simulink model "receiver_overall_v3"  (Simulink 7.5)
settings: Solver=FixedStepDiscrete  SolverMode=SingleTasking  StartTime=0.0  StopTime=(length(simin.signals.values)-1)/Fs  FixedStep=1  RelTol=1e-3
undefined symbols (not defined in the file): Fs
libraries: xbsIndex_r4 x939, symbols x8, dspsigops x2
(part 2 of 9)

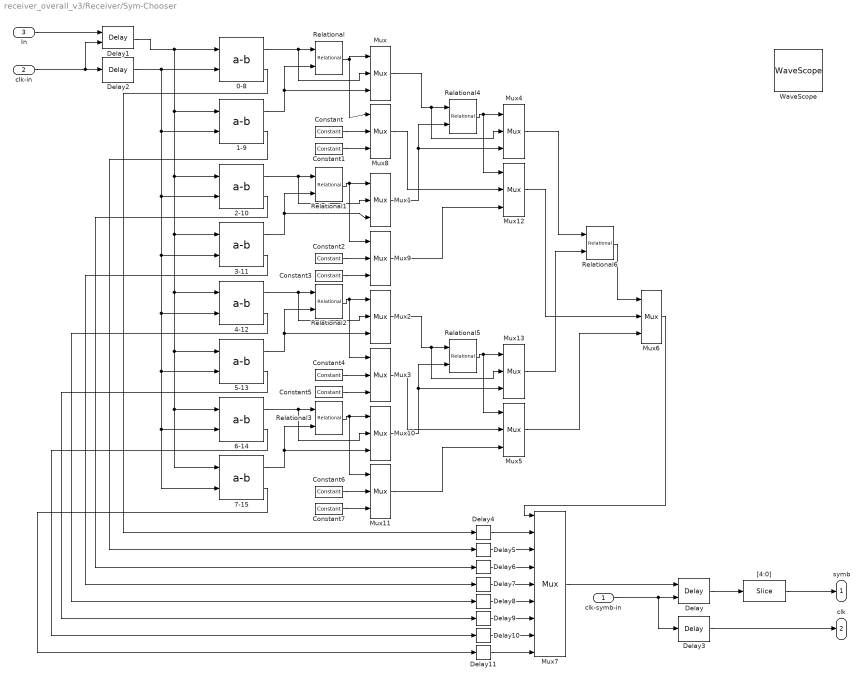
== system receiver_overall_v3/Receiver/Sym-Chooser ==
  clk-symb-in : Inport
  clk-in : Inport  Port=2
  In : Inport  Port=3
  0-8 : symbols/a-b  SystemSampleTime=-1  a=0  b=8  chip_a=1618456172
  1-9 : symbols/a-b  SystemSampleTime=-1  a=1  b=9  chip_a=1309113062
  2-10 : symbols/a-b  SystemSampleTime=-1  a=2  b=10  chip_a=1826650030
  3-11 : symbols/a-b  SystemSampleTime=-1  a=3  b=11  chip_a=1724778362
  4-12 : symbols/a-b  SystemSampleTime=-1  a=4  b=12  chip_a=778887287
  5-13 : symbols/a-b  SystemSampleTime=-1  a=5  b=13  chip_a=2061946375
  6-14 : symbols/a-b  SystemSampleTime=-1  a=6  b=14  chip_a=2007919840
  7-15 : symbols/a-b  SystemSampleTime=-1  a=7  b=15  chip_a=125494990
  Constant : xbsIndex_r4/Constant  arith_type=Unsigned  const=0  n_bits=3  bin_pt=0  explicit_period=off  period=1  equ=P=C  opselect=C  inp2=PCIN>>17  opr=+  inp1=P  carry=CIN  dbl_ovrd=off  block_type=constant
      settings: block_version=12.2
  Constant1 : xbsIndex_r4/Constant  arith_type=Unsigned  const=1  n_bits=3  bin_pt=0  explicit_period=off  period=1  equ=P=C  opselect=C  inp2=PCIN>>17  opr=+  inp1=P  carry=CIN  dbl_ovrd=off  block_type=constant
      settings: block_version=12.2
  Constant2 : xbsIndex_r4/Constant  arith_type=Unsigned  const=2  n_bits=3  bin_pt=0  explicit_period=off  period=1  equ=P=C  opselect=C  inp2=PCIN>>17  opr=+  inp1=P  carry=CIN  dbl_ovrd=off  block_type=constant
      settings: block_version=12.2
  Constant3 : xbsIndex_r4/Constant  arith_type=Unsigned  const=3  n_bits=3  bin_pt=0  explicit_period=off  period=1  equ=P=C  opselect=C  inp2=PCIN>>17  opr=+  inp1=P  carry=CIN  dbl_ovrd=off  block_type=constant
      settings: block_version=12.2
  Constant4 : xbsIndex_r4/Constant  arith_type=Unsigned  const=4  n_bits=3  bin_pt=0  explicit_period=off  period=1  equ=P=C  opselect=C  inp2=PCIN>>17  opr=+  inp1=P  carry=CIN  dbl_ovrd=off  block_type=constant
      settings: block_version=12.2
  Constant5 : xbsIndex_r4/Constant  arith_type=Unsigned  const=5  n_bits=3  bin_pt=0  explicit_period=off  period=1  equ=P=C  opselect=C  inp2=PCIN>>17  opr=+  inp1=P  carry=CIN  dbl_ovrd=off  block_type=constant
      settings: block_version=12.2
  Constant6 : xbsIndex_r4/Constant  arith_type=Unsigned  const=6  n_bits=3  bin_pt=0  explicit_period=off  period=1  equ=P=C  opselect=C  inp2=PCIN>>17  opr=+  inp1=P  carry=CIN  dbl_ovrd=off  block_type=constant
      settings: block_version=12.2
  Constant7 : xbsIndex_r4/Constant  arith_type=Unsigned  const=7  n_bits=3  bin_pt=0  explicit_period=off  period=1  equ=P=C  opselect=C  inp2=PCIN>>17  opr=+  inp1=P  carry=CIN  dbl_ovrd=off  block_type=constant
      settings: block_version=12.2
  Delay : xbsIndex_r4/Delay  en=on  latency=1  dbl_ovrd=off  reg_retiming=off  block_type=delay
      settings: block_version=12.2
  Delay1 : xbsIndex_r4/Delay  en=on  latency=1  dbl_ovrd=off  reg_retiming=off  block_type=delay
      settings: block_version=12.2
  Delay{2..11} (10 alike) : xbsIndex_r4/Delay  en=off  latency=1  dbl_ovrd=off  reg_retiming=off  block_type=delay
      settings: block_version=12.2
  Mux{,1..3,6,8..11} (9 alike) : xbsIndex_r4/Mux  inputs=2  en=off  latency=0  precision=Full  arith_type=Unsigned  n_bits=16  bin_pt=14  quantization=Truncate  overflow=Wrap  dbl_ovrd=off  block_type=mux
      settings: block_version=12.2
  Mux{4..5,12..13} (4 alike) : xbsIndex_r4/Mux  inputs=2  en=off  latency=1  precision=Full  arith_type=Unsigned  n_bits=16  bin_pt=14  quantization=Truncate  overflow=Wrap  dbl_ovrd=off  block_type=mux
      settings: block_version=12.2
  Mux7 : xbsIndex_r4/Mux  inputs=8  en=off  latency=0  precision=Full  arith_type=Unsigned  n_bits=16  bin_pt=14  quantization=Truncate  overflow=Wrap  dbl_ovrd=off  block_type=mux
      settings: block_version=12.2
  Relational{,1..6} (7 alike) : xbsIndex_r4/Relational  mode=a<b  en=off  latency=0  dbl_ovrd=off  block_type=relational
      settings: block_version=12.2
  WaveScope : xbsIndex_r4/WaveScope  block_type=wavescope
      settings: block_version=12.2
  "[4:0]" : xbsIndex_r4/Slice  nbits=4  boolean_output=off  mode=Lower Bit Location + Width  bit1=0  base1=MSB of Input  bit0=0  base0=LSB of Input  dbl_ovrd=off  block_type=slice
      settings: block_version=12.1
  symb : Outport
  clk : Outport  Port=2
  wires:
  "[4:0]"/1 -> symb/1
  Delay1/1 -> 0-8/1, 1-9/1, 2-10/1, 3-11/1, 4-12/1, 5-13/1, 7-15/1, 6-14/1
  Relational/1 -> Mux/1, Mux8/1
  0-8/1 -> Relational/1, Mux/2
  1-9/1 -> Relational/2, Mux/3
  0-8/2 -> Delay4/1
  1-9/2 -> Delay5/1
  2-10/2 -> Delay6/1
  3-11/2 -> Delay7/1
  4-12/2 -> Delay8/1
  5-13/2 -> Delay9/1
  6-14/2 -> Delay10/1
  7-15/2 -> Delay11/1
  Constant/1 -> Mux8/2
  Constant1/1 -> Mux8/3
  Relational1/1 -> Mux1/1, Mux9/1
  2-10/1 -> Relational1/1, Mux1/2
  3-11/1 -> Relational1/2, Mux1/3
  Constant2/1 -> Mux9/2
  Constant3/1 -> Mux9/3
  Relational2/1 -> Mux2/1, Mux3/1
  4-12/1 -> Relational2/1, Mux2/2
  5-13/1 -> Mux2/3, Relational2/2
  Constant4/1 -> Mux3/2
  Constant5/1 -> Mux3/3
  Relational3/1 -> Mux10/1, Mux11/1
  6-14/1 -> Relational3/1, Mux10/2
  7-15/1 -> Relational3/2, Mux10/3
  Constant6/1 -> Mux11/2
  Constant7/1 -> Mux11/3
  Relational4/1 -> Mux4/1, Mux12/1
  Mux/1 -> Relational4/1, Mux4/2
  Mux1/1 -> Relational4/2, Mux4/3
  Mux8/1 -> Mux12/2
  Mux9/1 -> Mux12/3
  Relational5/1 -> Mux13/1, Mux5/1
  Mux2/1 -> Relational5/1, Mux13/2
  Mux10/1 -> Relational5/2, Mux13/3
  Mux3/1 -> Mux5/2
  Mux11/1 -> Mux5/3
  Relational6/1 -> Mux6/1
  Mux4/1 -> Relational6/1
  Mux13/1 -> Relational6/2
  Mux12/1 -> Mux6/2
  Mux5/1 -> Mux6/3
  clk-in/1 -> Delay1/2, Delay2/1
  Mux7/1 -> Delay/1
  Delay/1 -> "[4:0]"/1
  clk-symb-in/1 -> Delay/2, Delay3/1
  Mux6/1 -> Mux7/1
  In/1 -> Delay1/1
  Delay4/1 -> Mux7/2
  Delay5/1 -> Mux7/3
  Delay6/1 -> Mux7/4
  Delay7/1 -> Mux7/5
  Delay8/1 -> Mux7/6
  Delay9/1 -> Mux7/7
  Delay10/1 -> Mux7/8
  Delay11/1 -> Mux7/9
  Delay2/1 -> 0-8/2, 6-14/2, 7-15/2, 5-13/2, 4-12/2, 3-11/2, 2-10/2, 1-9/2
  Delay3/1 -> clk/1

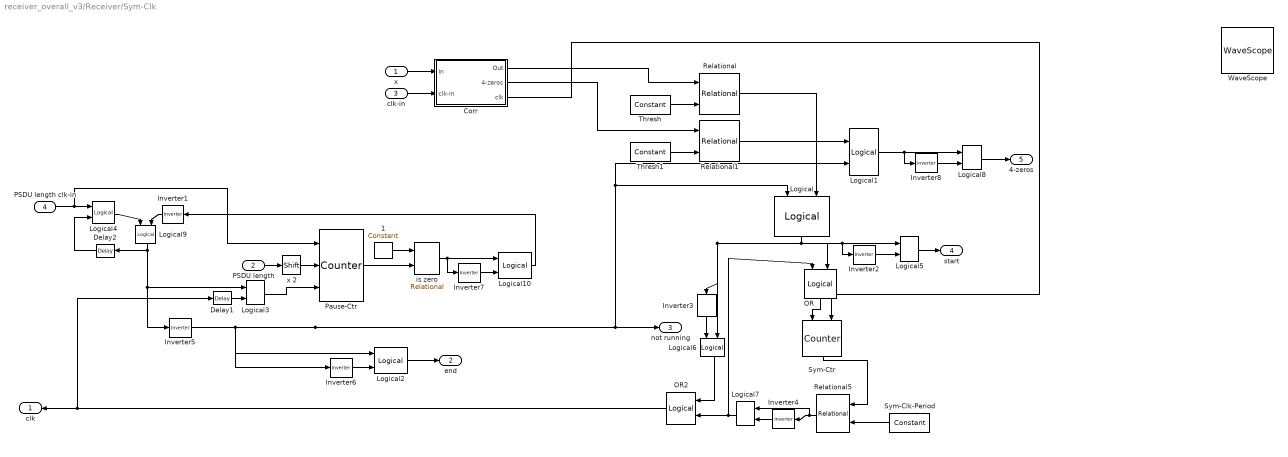
== system receiver_overall_v3/Receiver/Sym-Clk ==
  x : Inport
  PSDU length : Inport  Port=2  OutDataType=fixdt(1, 16)  OutScaling=2^0
  clk-in : Inport  Port=3
  PSDU length clk-in : Inport  Port=4  OutDataType=fixdt(1, 16)  OutScaling=2^0
  1 : xbsIndex_r4/Constant  arith_type=Unsigned  const=0  n_bits=1  bin_pt=0  explicit_period=off  period=1  equ=P=C  opselect=C  inp2=PCIN>>17  opr=+  inp1=P  carry=CIN  dbl_ovrd=off  block_type=constant
      settings: block_version=12.1
  Corr : Subsystem
  Delay1 : xbsIndex_r4/Delay  en=off  latency=3  dbl_ovrd=off  reg_retiming=off  block_type=delay
      settings: block_version=12.2
  Delay2 : xbsIndex_r4/Delay  en=off  latency=1  dbl_ovrd=off  reg_retiming=off  block_type=delay
      settings: block_version=12.2
  Inverter{1..4,6..8} (7 alike) : xbsIndex_r4/Inverter  en=off  latency=1  dbl_ovrd=off  block_type=inv
      settings: block_version=12.2
  Inverter5 : xbsIndex_r4/Inverter  en=off  latency=0  dbl_ovrd=off  block_type=inv
      settings: block_version=12.2
  Logical{,1..3,5..10} (10 alike) : xbsIndex_r4/Logical  logical_function=AND  inputs=2  en=off  latency=0  precision=Full  arith_type=Unsigned  n_bits=16  bin_pt=0  align_bp=on  dbl_ovrd=off  block_type=logical
      Logical settings: xl_area=[1 0 0 2 0 0 0]  block_version=12.1
      Logical1 settings: xl_area=[1 0 0 2 0 0 0]  block_version=12.1
      Logical10 settings: block_version=12.2
      Logical2 settings: block_version=12.2
      Logical3 settings: block_version=12.2
      Logical5 settings: block_version=12.2
      Logical6 settings: block_version=12.2
      Logical7 settings: block_version=12.2
      Logical8 settings: block_version=12.2
      Logical9 settings: block_version=12.2
  Logical4 : xbsIndex_r4/Logical  logical_function=OR  inputs=2  en=off  latency=0  precision=Full  arith_type=Unsigned  n_bits=16  bin_pt=0  align_bp=on  dbl_ovrd=off  block_type=logical
      settings: block_version=12.2
  OR : xbsIndex_r4/Logical  logical_function=OR  inputs=2  en=off  latency=0  precision=Full  arith_type=Unsigned  n_bits=16  bin_pt=0  align_bp=on  dbl_ovrd=off  block_type=logical
      settings: xl_area=[1 0 0 1 0 0 0]  block_version=12.1
  OR2 : xbsIndex_r4/Logical  logical_function=OR  inputs=2  en=off  latency=0  precision=Full  arith_type=Unsigned  n_bits=16  bin_pt=0  align_bp=on  dbl_ovrd=off  block_type=logical
      settings: xl_area=[1 0 0 1 0 0 0]  block_version=12.1
  Pause-Ctr : xbsIndex_r4/Counter  cnt_type=Free Running  cnt_to=Inf  operation=Down  start_count=0  cnt_by_val=1  arith_type=Unsigned  n_bits=13  bin_pt=0  load_pin=on  rst=off  en=on  explicit_period=off  period=1600  dbl_ovrd=off  use_behavioral_HDL=off  implementation=Fabric  block_type=counter
      settings: block_version=12.2
  Relational : xbsIndex_r4/Relational  mode=a>b  en=off  latency=0  dbl_ovrd=off  block_type=relational
      settings: xl_area=[4 0 0 7 0 0 0]  block_version=12.1
  Relational1 : xbsIndex_r4/Relational  mode=a>b  en=off  latency=0  dbl_ovrd=off  block_type=relational
      settings: xl_area=[4 0 0 7 0 0 0]  block_version=12.1
  Relational5 : xbsIndex_r4/Relational  mode=a=b  en=off  latency=1  dbl_ovrd=off  block_type=relational
      settings: xl_area=[2 0 0 4 0 0 0]  block_version=12.1
  Sym-Clk-Period : xbsIndex_r4/Constant  arith_type=Unsigned  const=32  n_bits=6  bin_pt=0  explicit_period=off  period=1  equ=P=C  opselect=C  inp2=PCIN>>17  opr=+  inp1=P  carry=CIN  dbl_ovrd=off  block_type=constant
      settings: block_version=12.1
  Sym-Ctr : xbsIndex_r4/Counter  cnt_type=Free Running  cnt_to=0  operation=Up  start_count=0  cnt_by_val=1  arith_type=Unsigned  n_bits=8  bin_pt=0  load_pin=off  rst=on  en=on  explicit_period=off  period=1  dbl_ovrd=off  use_behavioral_HDL=off  implementation=Fabric  block_type=counter
      settings: xl_area=[5 8 0 8 0 0 0]  block_version=12.1
  Thresh : xbsIndex_r4/Constant  arith_type=Unsigned  const=80  n_bits=7  bin_pt=0  explicit_period=off  period=1  equ=P=C  opselect=C  inp2=PCIN>>17  opr=+  inp1=P  carry=CIN  dbl_ovrd=off  block_type=constant
      settings: block_version=12.1
  Thresh1 : xbsIndex_r4/Constant  arith_type=Unsigned  const=80  n_bits=7  bin_pt=0  explicit_period=off  period=1  equ=P=C  opselect=C  inp2=PCIN>>17  opr=+  inp1=P  carry=CIN  dbl_ovrd=off  block_type=constant
      settings: block_version=12.1
  WaveScope : xbsIndex_r4/WaveScope  block_type=wavescope
      settings: block_version=12.2
  is zero : xbsIndex_r4/Relational  mode=a=b  en=off  latency=0  dbl_ovrd=off  block_type=relational
      settings: block_version=12.2
  x 2 : xbsIndex_r4/Shift  shift_dir=Left  shift_bits=1  en=off  latency=0  precision=User Defined  arith_type=Unsigned  n_bits=13  bin_pt=0  quantization=Truncate  overflow=Wrap  dbl_ovrd=off  block_type=shift
      settings: block_version=12.2
  clk : Outport  OutDataType=fixdt(1, 16)  OutScaling=2^0
  end : Outport  Port=2  OutDataType=fixdt(1, 16)  OutScaling=2^0
  not running : Outport  Port=3  OutDataType=fixdt(1, 16)  OutScaling=2^0
  start : Outport  Port=4  OutDataType=fixdt(1, 16)  OutScaling=2^0
  4-zeros : Outport  Port=5  OutDataType=fixdt(1, 16)  OutScaling=2^0
  wires:
  Thresh/1 -> Relational/2
  Relational/1 -> Logical/2
  Logical/1 -> OR/2, Logical5/1, Inverter2/1, Inverter3/1, Logical6/2
  x/1 -> Corr/1(In)
  OR/1 -> Sym-Ctr/1
  Inverter5/1 -> not running/1, Logical/1, Logical1/2, Logical2/1, Inverter6/1
  Logical2/1 -> end/1
  Sym-Ctr/1 -> Relational5/1
  Inverter6/1 -> Logical2/2
  Sym-Clk-Period/1 -> Relational5/2
  OR2/1 -> clk/1, Delay1/1
  Thresh1/1 -> Relational1/2
  Relational1/1 -> Logical1/1
  clk-in/1 -> Corr/2(clk-in)
  Corr/2(4-zeros) -> Relational1/1
  Logical5/1 -> start/1
  Inverter2/1 -> Logical5/2
  Corr/1(Out) -> Relational/1
  Corr/3(clk) -> Sym-Ctr/2
  Inverter3/1 -> Logical6/1
  Logical6/1 -> OR2/1
  Inverter4/1 -> Logical7/2
  Relational5/1 -> Inverter4/1, Logical7/1
  Logical7/1 -> OR2/2, OR/1
  Delay2/1 -> Logical4/2
  Logical4/1 -> Logical9/1
  Inverter1/1 -> Logical9/2
  Logical9/1 -> Delay2/1, Logical3/1, Inverter5/1
  x 2/1 -> Pause-Ctr/2
  PSDU length/1 -> x 2/1
  PSDU length clk-in/1 -> Logical4/1, Pause-Ctr/1
  Logical3/1 -> Pause-Ctr/3
  1/1 -> is zero/1
  Pause-Ctr/1 -> is zero/2
  Inverter7/1 -> Logical10/2
  is zero/1 -> Inverter7/1, Logical10/1
  Logical10/1 -> Inverter1/1
  Delay1/1 -> Logical3/2
  Logical1/1 -> Logical8/1, Inverter8/1
  Inverter8/1 -> Logical8/2
  Logical8/1 -> 4-zeros/1

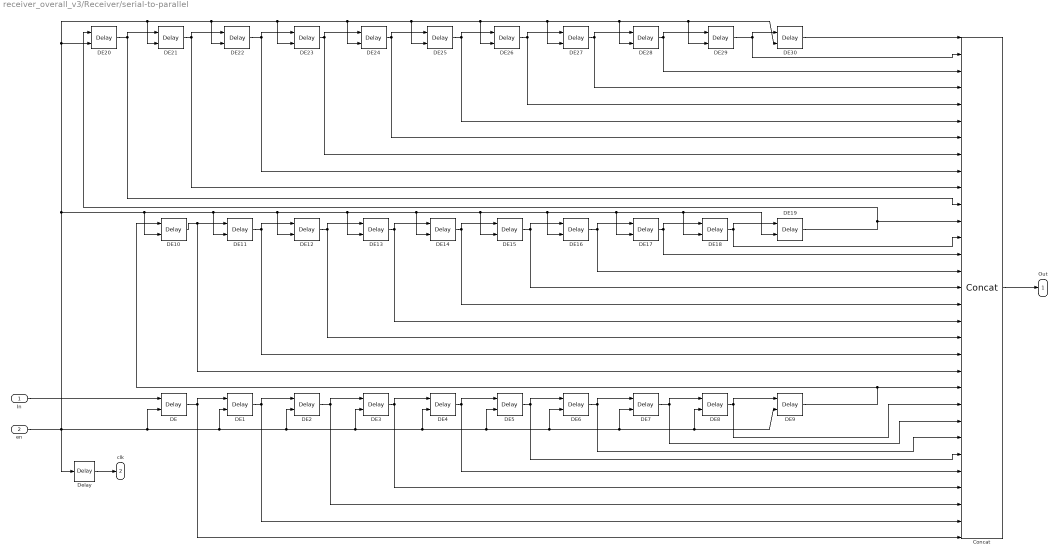
== system receiver_overall_v3/Receiver/serial-to-parallel ==
  In : Inport
  en : Inport  Port=2
  Concat : xbsIndex_r4/Concat  num_inputs=31  dbl_ovrd=off  block_type=concat
      settings: block_version=12.1
  DE{,1..30} (31 alike) : xbsIndex_r4/Delay  en=on  latency=1  dbl_ovrd=off  reg_retiming=off  block_type=delay
      settings: xl_area=[1 1 0 0 0 0 0]  block_version=12.1
  Delay : xbsIndex_r4/Delay  en=off  latency=1  dbl_ovrd=off  reg_retiming=off  block_type=delay
      settings: block_version=12.2
  Out : Outport
  clk : Outport  Port=2
  wires:
  In/1 -> DE/1
  en/1 -> DE20/2, DE21/2, DE22/2, DE23/2, DE24/2, DE25/2, DE26/2, DE27/2, DE28/2, DE30/2, DE29/2, DE19/2, DE18/2, DE17/2, DE16/2, DE15/2, DE14/2, DE13/2, DE12/2, DE11/2, DE10/2, DE1/2, DE2/2, DE3/2, DE4/2, DE5/2, DE6/2, DE7/2, DE8/2, DE9/2, DE/2, Delay/1
  DE/1 -> DE1/1, Concat/31
  DE1/1 -> DE2/1, Concat/30
  DE2/1 -> DE3/1, Concat/29
  DE3/1 -> DE4/1, Concat/28
  DE4/1 -> DE5/1, Concat/27
  DE5/1 -> DE6/1, Concat/26
  DE6/1 -> DE7/1, Concat/25
  DE8/1 -> DE9/1, Concat/23
  DE10/1 -> DE11/1, Concat/21
  DE11/1 -> DE12/1, Concat/20
  DE12/1 -> DE13/1, Concat/19
  DE13/1 -> DE14/1, Concat/18
  DE14/1 -> DE15/1, Concat/17
  DE15/1 -> DE16/1, Concat/16
  DE16/1 -> DE17/1, Concat/15
  DE17/1 -> DE18/1, Concat/14
  DE18/1 -> DE19/1, Concat/13
  DE20/1 -> DE21/1, Concat/11
  DE21/1 -> DE22/1, Concat/10
  DE22/1 -> DE23/1, Concat/9
  DE23/1 -> DE24/1, Concat/8
  DE24/1 -> DE25/1, Concat/7
  DE25/1 -> DE26/1, Concat/6
  DE26/1 -> DE27/1, Concat/5
  DE27/1 -> DE28/1, Concat/4
  DE28/1 -> DE29/1, Concat/3
  DE7/1 -> DE8/1, Concat/24
  DE29/1 -> DE30/1, Concat/2
  DE30/1 -> Concat/1
  DE19/1 -> Concat/12, DE20/1
  DE9/1 -> Concat/22, DE10/1
  Concat/1 -> Out/1
  Delay/1 -> clk/1

== system receiver_overall_v3/Receiver/to octet ==
  In : Inport
  clk-in : Inport  Port=2
  Concat : xbsIndex_r4/Concat  num_inputs=2  dbl_ovrd=off  block_type=concat
      settings: block_version=12.2
  Delay : xbsIndex_r4/Delay  en=on  latency=1  dbl_ovrd=off  reg_retiming=off  block_type=delay
      settings: block_version=12.2
  Delay1 : xbsIndex_r4/Delay  en=off  latency=1  dbl_ovrd=off  reg_retiming=off  block_type=delay
      settings: block_version=12.2
  Delay2 : xbsIndex_r4/Delay  en=off  latency=1  dbl_ovrd=off  reg_retiming=off  block_type=delay
      settings: block_version=12.2
  data : Outport
  clk : Outport  Port=2
  wires:
  Concat/1 -> data/1
  In/1 -> Delay1/1
  Delay1/1 -> Delay/1, Concat/1
  clk-in/1 -> Delay/2, Delay2/1
  Delay/1 -> Concat/2
  Delay2/1 -> clk/1

== system receiver_overall_v3/Receiver/FM demod/AGC ==
  I : Inport
  Q : Inport  Port=2
  CORDIC DIVIDER : Subsystem  mask(Xilinx CORDIC Divider){stages=8, num_width=22, num_binpt=19, pipeline_x=[1 1 1 1 1 1 1 1], prev_stages=8, pipeline=[1  1  1  1  1  1  1  1], prev_bits=21}
      mask prompts: stages "Number of Processing Elements (integer value starting from 1)"; num_width "X, Y, Data Width"; num_binpt "X,Y Binary Point Position"; pipeline_x "Latency for each Processing Element [1 0 0 1]"; prev_stages "Previous Number of Stages"; pipeline "Previous Pipeline Value"; prev_bits "Previous Number of Bits"
      mask help: This design implements a divider circuit using a fully parallel CORDIC (COordinate Rotation DIgital Computer) algorithm in linear vectoring mode with pre and post compensation. Using pre and post compensation techniques, this design can compute any arbitrary ratio y/x.
      mask init:
      | [bg,fg] = xlcmap('XBlock',0);
      | iPos = get_param(gcb,'Position');
      | iWidth=iPos(3)-iPos(1); iHeight=iPos(4)-iPos(2);
      | iCx=iWidth/2;
      | iCy=iHeight/2;
      | [logoX, logoY] = xlogo(iPos);
      | sav_gcb=gcb;
      | stages = round(sum(abs(stages)));
      | if (stages == 0)
      | 	stages = prev_stages;
      | end
      | x = zeros(1,stages);
      | pipe_size = max(size(pipeline_x));
      | if pipe_size >= stages
      | 	x(1,1:stages) = pipeline_x(1,1:stages);
      | else
      | 	x(1,1:pipe_size) = pipeline_x(1,1:pipe_size);
      | end
      | 
      | num_width = round(sum(abs(num_width)));
      | if (num_width < 2)
      | 	num_width = prev_bits;
      | end
      | 
      | if ((num_width-1) ~=prev_bits)
      |     % Draw the Normalization X Stage
      |     norm_x = find_system(sav_gcb, 'lookUnderMasks', 'all', 'FollowLinks','on','masktype', 'Normalize X');
      | 	a=find_system(norm_x{1}, 'lookUnderMasks', 'all', 'FollowLinks','on','masktype', 'Normalize Shift Stage');
      | 	for i= 2:length(a)
      | 		for j=1:3
      | 		    delete_line(norm_x{1}, ['Shift' int2str(i-1) '/' int2str(j)], ['Shift' int2str(i) '/' int2str(j)]);
      | 		end
      | 	end
      | 	delete_line(norm_x{1}, ['Shift' int2str(length(a)) '/1'],'norm/1');
      | 	delete_line(norm_x{1}, ['Shift' int2str(length(a)) '/2'],'shift/1');
      | 	delete_line(norm_x{1}, ['Shift' int2str(length(a)) '/3'],'Terminator1/1');
      | 	
      | 	for i=2:length(a)
      |       delete_block(a{i});
      | 	end
      | 	for i=2:(num_width-1),
      |         add_block([norm_x{1} '/Shift1'], [norm_x{1} '/Shift' int2str(i)],'position',[150+(i-1)*125, 70, 205+(i-1)*125, 130]);
      | 	end
      |     set_param([norm_x{1} '/' 'norm'], 'Position', [150+i*125, 72, 180+i*125, 86]);
      |     set_param([norm_x{1} '/' 'shift'], 'Position', [210+i*125, 92, 225+i*125, 108]);
      |     set_param([norm_x{1} '/' 'Terminator1'], 'Position', [240+i*125, 113, 270+i*125, 127]);
      |     for i= 2:(num_width-1)
      | 		for j=1:3
      | 		    add_line(norm_x{1}, ['Shift' int2str(i-1) '/' int2str(j)], ['Shift' int2str(i) '/' int2str(j)]);
      | 		end
      | 	end
      |     add_line(norm_x{1}, ['Shift' int2str((num_width-1)) '/1'],'norm/1');
      | 	add_line(norm_x{1}, ['Shift' int2str((num_width-1)) '/2'],'shift/1');
      | 	add_line(norm_x{1}, ['Shift' int2str((num_width-1)) '/3'],'Terminator1/1');
      |     
      |     % Draw the Normalization Y Stage
      |     norm_y = find_system(sav_gcb, 'lookUnderMasks', 'all', 'FollowLinks','on','masktype', 'Normalize Y');
      | 	a=find_system(norm_y{1}, 'lookUnderMasks', 'all', 'FollowLinks','on','masktype', 'Normalize Shift Stage');
      | 	for i= 2:length(a)
      | 		for j=1:3
      | 		    delete_line(norm_y{1}, ['Shift' int2str(i-1) '/' int2str(j)], ['Shift' int2str(i) '/' int2str(j)]);
      | 		end
      | 	end
      | 	delete_line(norm_y{1}, ['Shift' int2str(length(a)) '/1'],'norm/1');
      | 	delete_line(norm_y{1}, ['Shift' int2str(length(a)) '/2'],'shift/1');
      | 	delete_line(norm_y{1}, ['Shift' int2str(length(a)) '/3'],'Terminator1/1');
      | 	
      | 	for i=2:length(a)
      |       delete_block(a{i});
      | 	end
      | 	for i=2:(num_width-1)
      |         add_block([norm_y{1} '/Shift1'], [norm_y{1} '/Shift' int2str(i)],'position',[150+(i-1)*125, 70, 205+(i-1)*125, 130]);
      | 	end
      |     set_param([norm_y{1} '/' 'norm'], 'Position', [150+i*125, 72, 180+i*125, 86]);
      |     set_param([norm_y{1} '/' 'shift'], 'Position', [210+i*125, 92, 225+i*125, 108]);
      |     set_param([norm_y{1} '/' 'Terminator1'], 'Position', [240+i*125, 113, 270+i*125, 127]);
      |     for i= 2:(num_width-1)
      | 		for j=1:3
      | 		    add_line(norm_y{1}, ['Shift' int2str(i-1) '/' int2str(j)], ['Shift' int2str(i) '/' int2str(j)]);
      | 		end
      | 	end
      |     add_line(norm_y{1}, ['Shift' int2str((num_width-1)) '/1'],'norm/1');
      | 	add_line(norm_y{1}, ['Shift' int2str((num_width-1)) '/2'],'shift/1');
      | 	add_line(norm_y{1}, ['Shift' int2str((num_width-1)) '/3'],'Terminator1/1');
      | 	find_system(sav_gcb, 'lookUnderMasks', 'all', 'FollowLinks', 'on', 'MaskType','Xilinx Multiplexer Block');
      | 	set_param(sav_gcb, 'prev_bits',int2str((num_width-1)));
      | end
      | if (stages ~=prev_stages)
      | 	pipeline=x;
      |     iterative_divider = find_system(sav_gcb, 'lookUnderMasks', 'all', 'FollowLinks','on','masktype', 'CORDIC Iterative Divider');
      |   a=find_system(iterative_divider{1}, 'lookUnderMasks', 'all', 'FollowLinks','on','masktype', 'CORDIC iteration Divider');
      |   for i= 2:length(a)
      |     for j=1:3
      | 	  delete_line(iterative_divider{1}, ['CORDIC PE' int2str(i-1) '/' int2str(j)], ['CORDIC PE' int2str(i) '/' int2str(j)]);
      |     end
      |   end
      |   delete_line(iterative_divider{1}, ['CORDIC PE' int2str(length(a)) '/1'],'Terminator1/1');
      |   delete_line(iterative_divider{1}, ['CORDIC PE' int2str(length(a)) '/2'],'Terminator2/1');
      |   delete_line(iterative_divider{1}, ['CORDIC PE' int2str(length(a)) '/3'],'Z/1');
      |   for i=2:length(a)
      |      delete_block(a{i});
      |   end
      |   for i=2:stages,
      |       add_block([iterative_divider{1} '/CORDIC PE1'], [iterative_divider{1} '/CORDIC PE' int2str(i)], 'ii', int2str(i-1),'pipeline',['pipeline(1,' int2str(i) ')'],'position',[150+(i-1)*125, 70, 205+(i-1)*125, 130]);
      |   end
      |   for i= 2:stages,
      |      for j=1:3
      | 	     add_line(iterative_divider{1}, ['CORDIC PE' int2str(i-1) '/' int2str(j)], ['CORDIC PE' int2str(i) '/' int2str(j)], 'autorouting', 'on');
      |      end
      |   end
      |   set_param([iterative_divider{1} '/' 'Terminator1'], 'Position', [150+stages*125, 72, 180+stages*125, 86]);
      |   set_param([iterative_divider{1} '/' 'Terminator2'], 'Position', [210+stages*125, 92, 225+stages*125, 108]);
      |   set_param([iterative_divider{1} '/' 'Z'], 'Position', [240+stages*125, 113, 270+stages*125, 127]);
      | 
      |   add_line(iterative_divider{1}, ['CORDIC PE' int2str(stages) '/1'], 'Terminator1/1', 'autorouting', 'on');
      |   add_line(iterative_divider{1}, ['CORDIC PE' int2str(stages) '/2'], 'Terminator2/1', 'autorouting', 'on');
      |   add_line(iterative_divider{1}, ['CORDIC PE' int2str(stages) '/3'],'Z/1', 'autorouting', 'on');
      |    % force a "compile" of the constituent constant blocks to
      |    % workaround a data propagation problem
      |    find_system(iterative_divider{1}, 'lookUnderMasks', 'all', 'FollowLinks', 'on', 'MaskType','Xilinx Constant Block');
      |    set_param(sav_gcb, 'prev_stages', int2str(stages));
      |    set_param(sav_gcb, 'pipeline', [ '[' int2str(x) ']']);
      | else
      | 	if (sum(pipeline~=x))
      | 		set_param(sav_gcb, 'pipeline', [ '[' int2str(x) ']']);
      | 	end
      | end
      | 
      | str = sprintf('-%d',sum(x) + num_width + 4);
      settings: CopyFcn=set_param(gcb, 'MaskSelfModifiable', 'on', 'LinkStatus', 'none');
      mask Help: eval('');xlDoc('-book','sysgen','-topic','CORDIC_DIVIDER');
      mask Display:
      | patch([0 iWidth iWidth 0],[0 0 iHeight iHeight] , bg);
      | patch(logoX,logoY , fg);
      | text(iCx-6,iCy,'z');
      | text(iCx,iCy+4,str);
      | port_label('input',1,'x');
      | port_label('input',2,'y');
      | port_label('output',1,'y/x');
      | plot([0 0 iWidth iWidth 0], [0 iHeight iHeight 0 0]);
  Convert : xbsIndex_r4/Convert  arith_type="Signed  (2's comp)"  n_bits=16  bin_pt=14  quantization=Truncate  overflow=Wrap  en=off  latency=0  dbl_ovrd=off  pipeline=off  block_type=convert
      settings: block_version=12.2
  Convert1 : xbsIndex_r4/Convert  arith_type="Signed  (2's comp)"  n_bits=16  bin_pt=14  quantization=Truncate  overflow=Wrap  en=off  latency=0  dbl_ovrd=off  pipeline=off  block_type=convert
      settings: block_version=12.2
  Moving Average : Subsystem
  Mult4 : xbsIndex_r4/Mult  precision=Full  arith_type="Signed  (2's comp)"  n_bits=16  bin_pt=14  quantization=Truncate  overflow=Wrap  en=off  latency=4  dbl_ovrd=off  use_behavioral_HDL=off  opt=Speed  use_embedded=off  optimum_pipeline=on  pipeline=on  use_rpm=on  placement_style=Triangular  block_type=mult
      settings: block_version=12.2
  Mult5 : xbsIndex_r4/Mult  precision=Full  arith_type="Signed  (2's comp)"  n_bits=16  bin_pt=14  quantization=Truncate  overflow=Wrap  en=off  latency=4  dbl_ovrd=off  use_behavioral_HDL=off  opt=Speed  use_embedded=off  optimum_pipeline=on  pipeline=on  use_rpm=on  placement_style=Triangular  block_type=mult
      settings: block_version=12.2
  level estimate : Subsystem
      mask Display:
      | port_label('input',1,'I');
      | port_label('input',2,'Q');
      | port_label('output',1,'\approx sqrt(I^2+Q^2)','texmode','on');
  reference : xbsIndex_r4/Constant  arith_type=Signed (2's comp)  const=1  n_bits=22  bin_pt=19  explicit_period=on  period=1  equ=P=C  opselect=C  inp2=PCIN>>17  opr=+  inp1=P  carry=CIN  dbl_ovrd=off  block_type=constant
      settings: block_version=12.2
  I' : Outport
  Q' : Outport  Port=2
  wires:
  level estimate/1(Out1) -> Moving Average/1(in)
  I/1 -> level estimate/1(In1), Mult4/1
  Q/1 -> level estimate/2(In2), Mult5/2
  Convert/1 -> I'/1
  Convert1/1 -> Q'/1
  reference/1 -> CORDIC DIVIDER/2(y)
  Moving Average/1(short) -> CORDIC DIVIDER/1(x)
  Mult4/1 -> Convert/1
  Mult5/1 -> Convert1/1
  CORDIC DIVIDER/1(div) -> Mult5/1, Mult4/2

== system receiver_overall_v3/Receiver/FM demod/CORDIC ATAN ==
  note: The CORDIC algorithm is implemented in 3 steps.
      |
      | Step 1: Coarse Angle Rotation.  The algorithm converges only for angles between -pi/2 and pi/2, so if x < zero, the input vector is reflected
      | to the 1st or 3rd quadrant by making the x-coordinate non-negative.
      |
      | Step 2: Fine Angle Rotation.  For rectangular-to-polar conversion, the resulting vector is rotated through progressively smaller angles, such that y goes
      | to zero. In the i-th stage, the angular rotation is by either +/- atan(1/2^i), depending on whether or not its input y is less than or greater than zero.
      |
      | Step 3: Angle Correction. If there was a reflection applied in Step 1, this step applies the appropriate angle correction by subtracting it from +/- pi.
  x : Inport  OutDataType=sfix(16)  OutScaling=2^0
  y : Inport  Port=2  OutDataType=sfix(16)  OutScaling=2^0
  CORDIC  Pipe Balance : xbsIndex_r4/Delay  en=off  latency=sum(pipeline)  dbl_ovrd=off  reg_retiming=off  block_type=delay
      settings: infoedit="Delay line having  configurable length.<P><P>Hardware notes: A delay line is a chain, each link of which is an SRL16 followed by a flip-flop. If register retiming is enabled, the delay line is a chain of flip-flops."  xl_area=[1 1 0 1 0 0 0]  block_version=VER_STRING_GOES_HERE
  CORDIC  Pipe Balance1 : xbsIndex_r4/Delay  en=off  latency=sum(pipeline)+1  dbl_ovrd=off  reg_retiming=off  block_type=delay
      settings: infoedit="Delay line having  configurable length.<P><P>Hardware notes: A delay line is a chain, each link of which is an SRL16 followed by a flip-flop. If register retiming is enabled, the delay line is a chain of flip-flops."  xl_area=[1 1 0 1 0 0 0]  block_version=VER_STRING_GOES_HERE
  CORDIC  Pipe Balance2 : xbsIndex_r4/Delay  en=off  latency=1  dbl_ovrd=off  reg_retiming=off  block_type=delay
      settings: infoedit="Delay line having  configurable length.<P><P>Hardware notes: A delay line is a chain, each link of which is an SRL16 followed by a flip-flop. If register retiming is enabled, the delay line is a chain of flip-flops."  xl_area=[17 33 0 0 0 0 0]  block_version=VER_STRING_GOES_HERE
  CORDIC Fine Angle PE : Subsystem  mask(CORDIC parallel PE){}
      mask init:
      | [bg,fg] = xlcmap('XBlock',0);
      | iPos = get_param(gcb,'Position');
      | iWidth=iPos(3)-iPos(1); iHeight=iPos(4)-iPos(2);
      | iCx=iWidth/2;
      | iCy=iHeight/2;
      | [logoX, logoY] = xlogo(iPos);
      mask Display:
      | patch([0 iWidth iWidth 0],[0 0 iHeight iHeight] , bg);
      | patch(logoX,logoY , fg);
      | port_label('input',1,'x');
      | port_label('input',2,'y');
      | port_label('input',3,'z');
      | port_label('output',1,'X');
      | port_label('output',2,'Z');
      | plot([0 0 iWidth iWidth 0], [0 iHeight iHeight 0 0]);
  Constant : xbsIndex_r4/Constant  arith_type=Signed (2's comp)  const=0  n_bits=pe_nbits  bin_pt=pe_binpt  explicit_period=off  period=1  equ=P=C  opselect=C  inp2=PCIN>>17  opr=+  inp1=P  carry=CIN  dbl_ovrd=off  block_type=constant
      settings: block_version=VER_STRING_GOES_HERE
  Quadrant Correct : Subsystem
      mask init:
      | [bg,fg] = xlcmap('XBlock',0);
      | iPos = get_param(gcb,'Position');
      | iWidth=iPos(3)-iPos(1); iHeight=iPos(4)-iPos(2);
      | iCx=iWidth/2;
      | iCy=iHeight/2;
      | [logoX, logoY] = xlogo(iPos);
      mask Display:
      | patch([0 iWidth iWidth 0],[0 0 iHeight iHeight] , bg);
      | patch(logoX,logoY , fg);
      | port_label('input',1,'Z in');
      | port_label('input',2,'sgn(y)');
      | port_label('input',3,'sgn(x)');
      | port_label('output',1,'Z');
      | plot([0 0 iWidth iWidth 0], [0 iHeight iHeight 0 0]);
  Quadrant Map : Subsystem
      mask init:
      | [bg,fg] = xlcmap('XBlock',0);
      | iPos = get_param(gcb,'Position');
      | iWidth=iPos(3)-iPos(1); iHeight=iPos(4)-iPos(2);
      | iCx=iWidth/2;
      | iCy=iHeight/2;
      | [logoX, logoY] = xlogo(iPos);
      mask Display:
      | patch([0 iWidth iWidth 0],[0 0 iHeight iHeight] , bg);
      | patch(logoX,logoY , fg);
      | port_label('input',1,'x');
      | port_label('input',2,'y');
      | port_label('output',1,'X');
      | port_label('output',2,'Y');
      | port_label('output',3,'sgn(y)');
      | port_label('output',4,'sgn(x)');
      | plot([0 0 iWidth iWidth 0], [0 iHeight iHeight 0 0]);
  X : Outport  OutDataType=sfix(16)  OutScaling=2^0
  Z : Outport  Port=2  OutDataType=sfix(16)  OutScaling=2^0
  wires:
  Constant/1 -> CORDIC Fine Angle PE/3(z)
  Quadrant Map/1(X) -> CORDIC Fine Angle PE/1(x)
  Quadrant Map/2(Y) -> CORDIC Fine Angle PE/2(y)
  x/1 -> Quadrant Map/1(x)
  y/1 -> Quadrant Map/2(y)
  Quadrant Map/3(sign(y)) -> CORDIC  Pipe Balance/1
  Quadrant Map/4(sign(x)) -> CORDIC  Pipe Balance1/1
  CORDIC  Pipe Balance/1 -> Quadrant Correct/2(PI_ addsub)
  CORDIC  Pipe Balance1/1 -> Quadrant Correct/3(Z MUX SEL)
  CORDIC Fine Angle PE/2(Z) -> Quadrant Correct/1(Z IN)
  Quadrant Correct/1(Z) -> Z/1
  CORDIC Fine Angle PE/1(X) -> CORDIC  Pipe Balance2/1
  CORDIC  Pipe Balance2/1 -> X/1

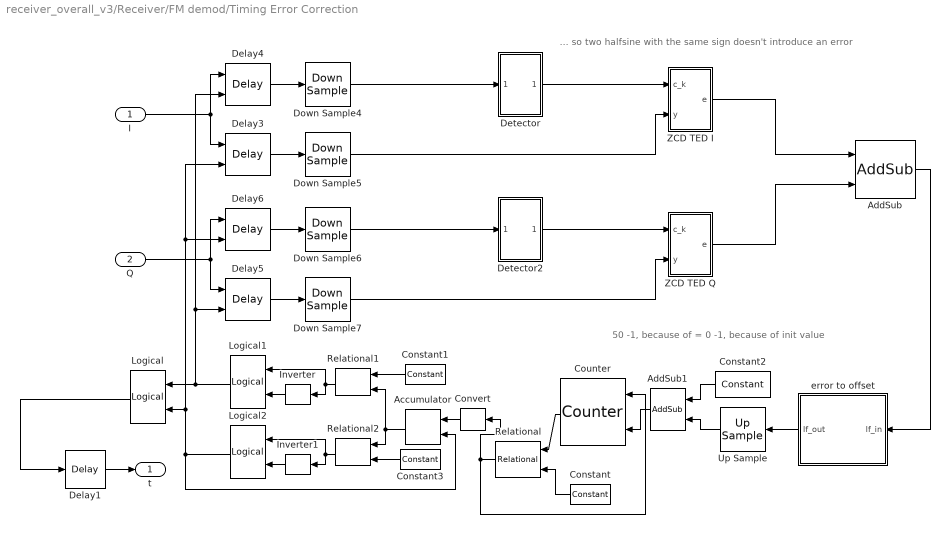
== system receiver_overall_v3/Receiver/FM demod/Timing Error Correction ==
  note: 50
      | -1, because of = 0
      | -1, because of init value
  note: ... so two halfsine with the same sign doesn't introduce an error
  I : Inport
  Q : Inport  Port=2
  Accumulator : xbsIndex_r4/Accumulator  operation=Add  n_bits=2  overflow=Wrap  scale=1  rst=on  hasbypass=off  en=off  dbl_ovrd=off  use_behavioral_HDL=on  implementation=Fabric  block_type=accum
      settings: block_version=12.2
  AddSub : xbsIndex_r4/AddSub  mode=Subtraction  use_carryin=off  use_carryout=off  en=off  latency=1  precision=Full  arith_type=Unsigned  n_bits=16  bin_pt=14  quantization=Truncate  overflow=Wrap  dbl_ovrd=off  use_behavioral_HDL=off  hw_selection=Fabric  pipelined=off  block_type=addsub
      settings: block_version=12.2
  AddSub1 : xbsIndex_r4/AddSub  mode=Addition  use_carryin=off  use_carryout=off  en=off  latency=1  precision=User Defined  arith_type=Unsigned  n_bits=8  bin_pt=0  quantization=Truncate  overflow=Wrap  dbl_ovrd=off  use_behavioral_HDL=off  hw_selection=Fabric  pipelined=off  block_type=addsub
      settings: block_version=12.2
  Constant : xbsIndex_r4/Constant  arith_type=Unsigned  const=0  n_bits=1  bin_pt=0  explicit_period=off  period=1  equ=P=C  opselect=C  inp2=PCIN>>17  opr=+  inp1=P  carry=CIN  dbl_ovrd=off  block_type=constant
      settings: block_version=12.2
  Constant1 : xbsIndex_r4/Constant  arith_type=Unsigned  const=1  n_bits=2  bin_pt=0  explicit_period=off  period=1  equ=P=C  opselect=C  inp2=PCIN>>17  opr=+  inp1=P  carry=CIN  dbl_ovrd=off  block_type=constant
      settings: block_version=12.2
  Constant2 : xbsIndex_r4/Constant  arith_type=Unsigned  const=48  n_bits=8  bin_pt=0  explicit_period=on  period=1  equ=P=C  opselect=C  inp2=PCIN>>17  opr=+  inp1=P  carry=CIN  dbl_ovrd=off  block_type=constant
      settings: block_version=12.2
  Constant3 : xbsIndex_r4/Constant  arith_type=Unsigned  const=2  n_bits=2  bin_pt=0  explicit_period=off  period=1  equ=P=C  opselect=C  inp2=PCIN>>17  opr=+  inp1=P  carry=CIN  dbl_ovrd=off  block_type=constant
      settings: block_version=12.2
  Convert : xbsIndex_r4/Convert  arith_type=Unsigned  n_bits=1  bin_pt=0  quantization=Truncate  overflow=Wrap  en=off  latency=0  dbl_ovrd=off  pipeline=off  block_type=convert
      settings: block_version=12.2
  Counter : xbsIndex_r4/Counter  cnt_type=Free Running  cnt_to=Inf  operation=Down  start_count=0  cnt_by_val=1  arith_type=Unsigned  n_bits=8  bin_pt=0  load_pin=on  rst=off  en=off  explicit_period=on  period=1  dbl_ovrd=off  use_behavioral_HDL=off  implementation=Fabric  block_type=counter
      settings: block_version=12.2
  Delay1 : xbsIndex_r4/Delay  en=off  latency=7  dbl_ovrd=off  reg_retiming=off  block_type=delay
      settings: block_version=12.2
  Delay{3..6} (4 alike) : xbsIndex_r4/Delay  en=on  latency=1  dbl_ovrd=off  reg_retiming=off  block_type=delay
      settings: block_version=12.2
  Detector : Subsystem
  Detector2 : Subsystem
  Down Sample{4..7} (4 alike) : xbsIndex_r4/Down Sample  sample_ratio=100  sample_phase=First Value of Frame  en=off  latency=0  dbl_ovrd=off  block_type=dsamp
      settings: xl_area=[1 1 0 0 0 0 0]  block_version=12.1
  Inverter : xbsIndex_r4/Inverter  en=off  latency=1  dbl_ovrd=off  block_type=inv
      settings: block_version=12.2
  Inverter1 : xbsIndex_r4/Inverter  en=off  latency=1  dbl_ovrd=off  block_type=inv
      settings: block_version=12.2
  Logical : xbsIndex_r4/Logical  logical_function=OR  inputs=2  en=off  latency=0  precision=Full  arith_type=Unsigned  n_bits=16  bin_pt=0  align_bp=on  dbl_ovrd=off  block_type=logical
      settings: block_version=12.2
  Logical1 : xbsIndex_r4/Logical  logical_function=AND  inputs=2  en=off  latency=0  precision=Full  arith_type=Unsigned  n_bits=16  bin_pt=0  align_bp=on  dbl_ovrd=off  block_type=logical
      settings: block_version=12.2
  Logical2 : xbsIndex_r4/Logical  logical_function=AND  inputs=2  en=off  latency=0  precision=Full  arith_type=Unsigned  n_bits=16  bin_pt=0  align_bp=on  dbl_ovrd=off  block_type=logical
      settings: block_version=12.2
  Relational : xbsIndex_r4/Relational  mode=a=b  en=off  latency=1  dbl_ovrd=off  block_type=relational
      settings: block_version=12.2
  Relational1 : xbsIndex_r4/Relational  mode=a=b  en=off  latency=1  dbl_ovrd=off  block_type=relational
      settings: block_version=12.2
  Relational2 : xbsIndex_r4/Relational  mode=a=b  en=off  latency=1  dbl_ovrd=off  block_type=relational
      settings: block_version=12.2
  Up Sample : xbsIndex_r4/Up Sample  sample_ratio=100  copy_samples=on  en=off  latency=0  dbl_ovrd=off  block_type=usamp
      settings: block_version=12.2
  ZCD TED I : Subsystem
  ZCD TED Q : Subsystem
  error to offset : Subsystem
      mask Display: disp('not a 2nd order\nLoop filter')
  t : Outport  OutDataType=fixdt(1, 16)  OutScaling=2^0
  wires:
  Relational2/1 -> Inverter1/1, Logical2/1
  Delay4/1 -> Down Sample4/1
  Delay3/1 -> Down Sample5/1
  Down Sample4/1 -> Detector/1(In1)
  Delay6/1 -> Down Sample6/1
  Delay5/1 -> Down Sample7/1
  Down Sample7/1 -> ZCD TED Q/2(y)
  Q/1 -> Delay6/1, Delay5/1
  I/1 -> Delay3/1, Delay4/1
  error to offset/1(lf_out) -> Up Sample/1
  Logical/1 -> Delay1/1
  Delay1/1 -> t/1
  Constant2/1 -> AddSub1/1
  Up Sample/1 -> AddSub1/2
  Constant/1 -> Relational/2
  Counter/1 -> Relational/1
  Relational/1 -> Convert/1, Counter/1
  AddSub1/1 -> Counter/2
  Convert/1 -> Accumulator/1
  Constant1/1 -> Relational1/1
  Accumulator/1 -> Relational1/2, Relational2/1
  Constant3/1 -> Relational2/2
  Logical1/1 -> Logical/1, Delay5/2, Delay4/2
  Relational1/1 -> Logical1/1, Inverter/1
  Inverter/1 -> Logical1/2
  Inverter1/1 -> Logical2/2
  Logical2/1 -> Logical/2, Delay6/2, Delay3/2, Accumulator/2
  Detector/1(Out1) -> ZCD TED I/1(c_k)
  Down Sample5/1 -> ZCD TED I/2(y)
  Down Sample6/1 -> Detector2/1(In1)
  Detector2/1(Out1) -> ZCD TED Q/1(c_k)
  ZCD TED I/1(e) -> AddSub/1
  ZCD TED Q/1(e) -> AddSub/2
  AddSub/1 -> error to offset/1(lf_in)

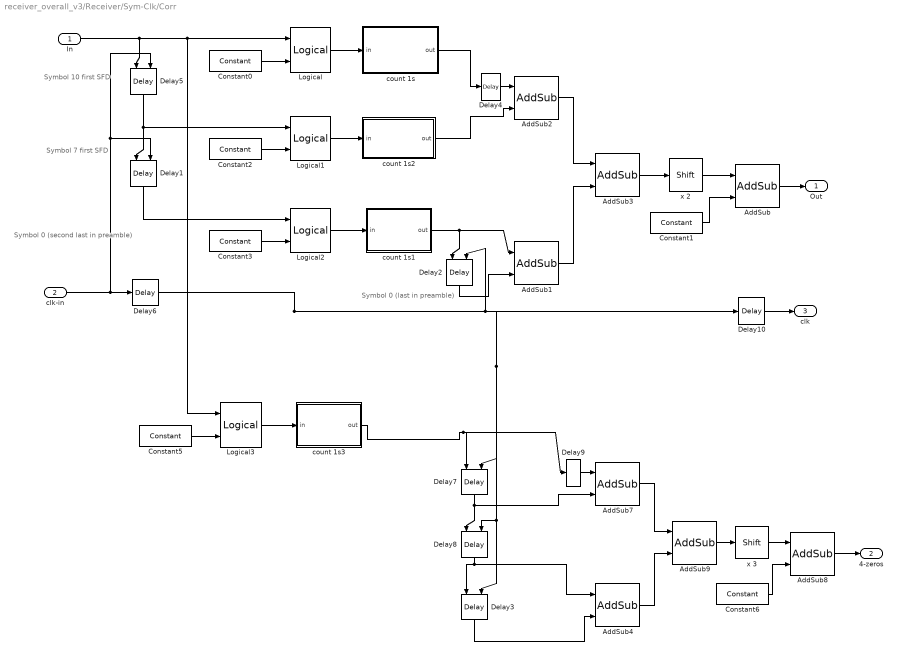
== system receiver_overall_v3/Receiver/Sym-Clk/Corr ==
  note: Symbol 0
      | (last in preamble)
  note: Symbol 0
      | (second last in preamble)
  note: Symbol 7
      | first SFD
  note: Symbol 10
      | first SFD
  In : Inport
  clk-in : Inport  Port=2
  AddSub : xbsIndex_r4/AddSub  mode=Subtraction  use_carryin=off  use_carryout=off  en=off  latency=1  precision=Full  arith_type=Unsigned  n_bits=16  bin_pt=14  quantization=Truncate  overflow=Wrap  dbl_ovrd=off  use_behavioral_HDL=off  hw_selection=Fabric  pipelined=off  block_type=addsub
      settings: xl_area=[4 0 0 6 0 0 0]  block_version=12.1
  AddSub{1..2,4,7} (4 alike) : xbsIndex_r4/AddSub  mode=Addition  use_carryin=off  use_carryout=off  en=off  latency=0  precision=Full  arith_type=Unsigned  n_bits=16  bin_pt=14  quantization=Truncate  overflow=Wrap  dbl_ovrd=off  use_behavioral_HDL=off  hw_selection=Fabric  pipelined=off  block_type=addsub
      settings: xl_area=[4 0 0 6 0 0 0]  block_version=12.1
  AddSub3 : xbsIndex_r4/AddSub  mode=Addition  use_carryin=off  use_carryout=off  en=off  latency=1  precision=Full  arith_type=Unsigned  n_bits=16  bin_pt=14  quantization=Truncate  overflow=Wrap  dbl_ovrd=off  use_behavioral_HDL=off  hw_selection=Fabric  pipelined=off  block_type=addsub
      settings: xl_area=[4 0 0 6 0 0 0]  block_version=12.1
  AddSub8 : xbsIndex_r4/AddSub  mode=Subtraction  use_carryin=off  use_carryout=off  en=off  latency=1  precision=Full  arith_type=Unsigned  n_bits=16  bin_pt=14  quantization=Truncate  overflow=Wrap  dbl_ovrd=off  use_behavioral_HDL=off  hw_selection=Fabric  pipelined=off  block_type=addsub
      settings: xl_area=[4 0 0 6 0 0 0]  block_version=12.1
  AddSub9 : xbsIndex_r4/AddSub  mode=Addition  use_carryin=off  use_carryout=off  en=off  latency=1  precision=Full  arith_type=Unsigned  n_bits=16  bin_pt=14  quantization=Truncate  overflow=Wrap  dbl_ovrd=off  use_behavioral_HDL=off  hw_selection=Fabric  pipelined=off  block_type=addsub
      settings: xl_area=[4 0 0 6 0 0 0]  block_version=12.1
  Constant0 : xbsIndex_r4/Constant  arith_type=Unsigned  const=320833617  n_bits=31  bin_pt=0  explicit_period=off  period=1/8  equ=P=C  opselect=C  inp2=PCIN>>17  opr=+  inp1=P  carry=CIN  dbl_ovrd=off  block_type=constant
      settings: block_version=12.1
  Constant1 : xbsIndex_r4/Constant  arith_type=Unsigned  const=124  n_bits=7  bin_pt=0  explicit_period=off  period=1/8  equ=P=C  opselect=C  inp2=PCIN>>17  opr=+  inp1=P  carry=CIN  dbl_ovrd=off  block_type=constant
      settings: block_version=12.1
  Constant2 : xbsIndex_r4/Constant  arith_type=Unsigned  const=125494990  n_bits=31  bin_pt=0  explicit_period=off  period=1/8  equ=P=C  opselect=C  inp2=PCIN>>17  opr=+  inp1=P  carry=CIN  dbl_ovrd=off  block_type=constant
      settings: block_version=12.1
  Constant3 : xbsIndex_r4/Constant  arith_type=Unsigned  const=1618456172  n_bits=31  bin_pt=0  explicit_period=off  period=1/8  equ=P=C  opselect=C  inp2=PCIN>>17  opr=+  inp1=P  carry=CIN  dbl_ovrd=off  block_type=constant
      settings: block_version=12.1
  Constant5 : xbsIndex_r4/Constant  arith_type=Unsigned  const=1618456172  n_bits=31  bin_pt=0  explicit_period=off  period=1/8  equ=P=C  opselect=C  inp2=PCIN>>17  opr=+  inp1=P  carry=CIN  dbl_ovrd=off  block_type=constant
      settings: block_version=12.1
  Constant6 : xbsIndex_r4/Constant  arith_type=Unsigned  const=124  n_bits=7  bin_pt=0  explicit_period=off  period=1/8  equ=P=C  opselect=C  inp2=PCIN>>17  opr=+  inp1=P  carry=CIN  dbl_ovrd=off  block_type=constant
      settings: block_version=12.1
  Delay{1..3,8} (4 alike) : xbsIndex_r4/Delay  en=on  latency=32  dbl_ovrd=off  reg_retiming=off  block_type=delay
      settings: block_version=12.2
  Delay10 : xbsIndex_r4/Delay  en=off  latency=3  dbl_ovrd=off  reg_retiming=off  block_type=delay
      settings: block_version=12.2
  Delay4 : xbsIndex_r4/Delay  en=off  latency=1  dbl_ovrd=off  reg_retiming=off  block_type=delay
      settings: block_version=12.2
  Delay5 : xbsIndex_r4/Delay  en=on  latency=33  dbl_ovrd=off  reg_retiming=off  block_type=delay
      settings: block_version=12.2
  Delay6 : xbsIndex_r4/Delay  en=off  latency=1  dbl_ovrd=off  reg_retiming=off  block_type=delay
      settings: block_version=12.2
  Delay7 : xbsIndex_r4/Delay  en=on  latency=33  dbl_ovrd=off  reg_retiming=off  block_type=delay
      settings: block_version=12.2
  Delay9 : xbsIndex_r4/Delay  en=off  latency=1  dbl_ovrd=off  reg_retiming=off  block_type=delay
      settings: block_version=12.2
  Logical{,1..3} (4 alike) : xbsIndex_r4/Logical  logical_function=XNOR  inputs=2  en=off  latency=0  precision=User Defined  arith_type=Unsigned  n_bits=32  bin_pt=0  align_bp=on  dbl_ovrd=off  block_type=logical
      settings: xl_area=[31 0 0 31 0 0 0]  block_version=12.1
  count 1s : Subsystem
  count 1s1 : Subsystem
  count 1s2 : Subsystem
  count 1s3 : Subsystem
  x 2 : xbsIndex_r4/Shift  shift_dir=Left  shift_bits=1  en=off  latency=0  precision=Full  arith_type=Unsigned  n_bits=7  bin_pt=0  quantization=Truncate  overflow=Wrap  dbl_ovrd=off  block_type=shift
      settings: xl_area=[0 0 0 0 0 0 0]  block_version=12.1
  x 3 : xbsIndex_r4/Shift  shift_dir=Left  shift_bits=1  en=off  latency=0  precision=Full  arith_type=Unsigned  n_bits=7  bin_pt=0  quantization=Truncate  overflow=Wrap  dbl_ovrd=off  block_type=shift
      settings: xl_area=[0 0 0 0 0 0 0]  block_version=12.1
  Out : Outport
  4-zeros : Outport  Port=2
  clk : Outport  Port=3
  wires:
  Constant0/1 -> Logical/2
  Logical/1 -> count 1s/1(in)
  Constant1/1 -> AddSub/2
  x 2/1 -> AddSub/1
  In/1 -> Delay5/1, Logical/1, Logical3/1
  AddSub/1 -> Out/1
  Delay5/1 -> Logical1/1, Delay1/1
  Constant2/1 -> Logical1/2
  Delay1/1 -> Logical2/1
  Constant3/1 -> Logical2/2
  Logical2/1 -> count 1s1/1(in)
  count 1s1/1(out) -> Delay2/1, AddSub1/1
  Logical1/1 -> count 1s2/1(in)
  Delay2/1 -> AddSub1/2
  count 1s/1(out) -> Delay4/1
  count 1s2/1(out) -> AddSub2/2
  AddSub2/1 -> AddSub3/1
  AddSub1/1 -> AddSub3/2
  AddSub3/1 -> x 2/1
  clk-in/1 -> Delay6/1, Delay5/2, Delay1/2
  Constant5/1 -> Logical3/2
  Logical3/1 -> count 1s3/1(in)
  Delay7/1 -> Delay8/1, AddSub7/2
  Delay8/1 -> Delay3/1, AddSub4/1
  Constant6/1 -> AddSub8/2
  x 3/1 -> AddSub8/1
  AddSub8/1 -> 4-zeros/1
  AddSub9/1 -> x 3/1
  Delay3/1 -> AddSub4/2
  AddSub7/1 -> AddSub9/1
  AddSub4/1 -> AddSub9/2
  Delay6/1 -> Delay2/2, Delay7/2, Delay3/2, Delay8/2, Delay10/1
  count 1s3/1(out) -> Delay7/1, Delay9/1
  Delay4/1 -> AddSub2/1
  Delay9/1 -> AddSub7/1
  Delay10/1 -> clk/1

== system receiver_overall_v3/Receiver/FM demod/AGC/CORDIC DIVIDER ==
  note: The CORDIC Divider algorithm is implemented in 4 steps.
      |
      | Step 1: Co-ordinate Rotation.  The CORDIC algorithm converges only for positive values of x, so if x < zero, the input vector is
      | reflected to the 1st or 3rd quadrant by making the x-coordinate non-negative. For normalizing X and Y, Y is always mapped to
      | a non-negative value. The Divider circuit has been designed to converge for all values of X and Y, except for the most negative value .
      |
      | Step 2: Normalization.  The CORDIC algorithm converges only for y <= 2 x. For  x > y, both the inputs X and Y are shifted to the
      | left till they have a 1 in the most significant bit (MSB).  The relative shift of Y over X is recorded and passed on to the Quadrant
      | Correct Stage.
      |
      | Step 3: Linear Rotations.  For ratio calculation, the resulting vector is rotated through progressively smaller angles, such that y goes
      | to zero. In the i-th stage, the rotation yields +/- y/x, depending on whether the input y is less than or greater than zero.
      |
      | Step 4: Co-ordinate Correction. If the axis was rotated Step 1 and a relative shift was applied to Y over X, this step assigns the appropriate
      | sign to the resulting ratio and multiplies it with 2^(relative_shift of Y over X).
  x : Inport  OutDataType=sfix(16)  OutScaling=2^0
  y : Inport  Port=2  OutDataType=sfix(16)  OutScaling=2^0
  Constant2 : xbsIndex_r4/Constant  arith_type=Signed (2's comp)  const=0  n_bits=stages+2  bin_pt=stages  explicit_period=off  period=1  equ=P=C  opselect=C  inp2=PCIN>>17  opr=+  inp1=P  carry=CIN  dbl_ovrd=off  block_type=constant
      settings: block_version=VER_STRING_GOES_HERE
  Delay : xbsIndex_r4/Delay  en=off  latency=sum(pipeline)  dbl_ovrd=off  reg_retiming=off  block_type=delay
      settings: infoedit="Delay line having  configurable length.<P><P>Hardware notes: A delay line is a chain, each link of which is an SRL16 followed by a flip-flop. If register retiming is enabled, the delay line is a chain of flip-flops."  xl_area=[1 1 0 1 0 0 0]  block_version=VER_STRING_GOES_HERE
  Delay1 : xbsIndex_r4/Delay  en=off  latency=sum(pipeline)  dbl_ovrd=off  reg_retiming=off  block_type=delay
      settings: infoedit="Delay line having  configurable length.<P><P>Hardware notes: A delay line is a chain, each link of which is an SRL16 followed by a flip-flop. If register retiming is enabled, the delay line is a chain of flip-flops."  xl_area=[2 4 0 4 0 0 0]  block_version=VER_STRING_GOES_HERE
  Iterative Divider : Subsystem  mask(CORDIC Iterative Divider){}
      mask init:
      | [bg,fg] = xlcmap('XBlock',0);
      | iPos = get_param(gcb,'Position');
      | iWidth=iPos(3)-iPos(1); iHeight=iPos(4)-iPos(2);
      | iCx=iWidth/2;
      | iCy=iHeight/2;
      | [logoX, logoY] = xlogo(iPos);
      mask Display:
      | patch([0 iWidth iWidth 0],[0 0 iHeight iHeight] , bg);
      | patch(logoX,logoY , fg);
      | port_label('input',1,'x');
      | port_label('input',2,'y');
      | port_label('input',3,'z');
      | port_label('output',1,'Z');
      | plot([0 0 iWidth iWidth 0], [0 iHeight iHeight 0 0]);
  Quadrant Correct : Subsystem  mask{num_width=num_width, num_binpt=num_binpt}
      mask prompts: num_width "Data Width"; num_binpt "Data Binary Point"
      mask init:
      | [bg,fg] = xlcmap('XBlock',0);
      | iPos = get_param(gcb,'Position');
      | iWidth=iPos(3)-iPos(1); iHeight=iPos(4)-iPos(2);
      | iCx=iWidth/2;
      | iCy=iHeight/2;
      | [logoX, logoY] = xlogo(iPos);
      mask Display:
      | patch([0 iWidth iWidth 0],[0 0 iHeight iHeight] , bg);
      | patch(logoX,logoY , fg);
      | port_label('input',1,'z');
      | port_label('input',2,'sign');
      | port_label('input',3,'norm');
      | port_label('output',1,'y/x');
      | plot([0 0 iWidth iWidth 0], [0 iHeight iHeight 0 0]);
  Quadrant Map : Subsystem  mask{num_width=num_width, num_binpt=num_binpt}
      mask prompts: num_binpt "Num_bin_pt"
      mask init:
      | [bg,fg] = xlcmap('XBlock',0);
      | iPos = get_param(gcb,'Position');
      | iWidth=iPos(3)-iPos(1); iHeight=iPos(4)-iPos(2);
      | iCx=iWidth/2;
      | iCy=iHeight/2;
      | [logoX, logoY] = xlogo(iPos);
      mask Display:
      | patch([0 iWidth iWidth 0],[0 0 iHeight iHeight] , bg);
      | patch(logoX,logoY , fg);
      | port_label('input',1,'x');
      | port_label('input',2,'y');
      | port_label('output',1,'norm_x');
      | port_label('output',2,'norm_y');
      | port_label('output',3,'sign');
      | port_label('output',4,'index');
      | plot([0 0 iWidth iWidth 0], [0 iHeight iHeight 0 0]);
  div : Outport  OutDataType=sfix(16)  OutScaling=2^0
  wires:
  Quadrant Correct/1(Z) -> div/1
  y/1 -> Quadrant Map/2(y)
  x/1 -> Quadrant Map/1(x)
  Delay1/1 -> Quadrant Correct/3(norm)
  Quadrant Map/4(index) -> Delay1/1
  Delay/1 -> Quadrant Correct/2(sign)
  Quadrant Map/3(sign) -> Delay/1
  Iterative Divider/1(Z) -> Quadrant Correct/1(z)
  Quadrant Map/2(norm_Y) -> Iterative Divider/2(y)
  Quadrant Map/1(norm_X) -> Iterative Divider/1(x)
  Constant2/1 -> Iterative Divider/3(z)
